simulink model "Messages1"  (R2020a)
settings: Solver=VariableStepAuto  StartTime=0.0  StopTime=0.3  RelTol=1e-3
settings Model: Creator=86188  LastModifiedBy=bzhan
settings DataIOCC: ReturnWorkspaceOutputs=off
settings DebuggingCC: ArithmeticOperatorsInVariantConditions=warning
settings SFSimCC: SimUseLocalCustomCode=off  CustomCodeUndefinedFunction=UseInterfaceOnly
settings RTWCC: RTWUseLocalCustomCode=off

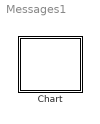
== system Messages1 ==
  Chart : Stateflow chart  TreatAsAtomicUnit=on

== stateflow chart Messages1/Chart ==
  state A
    en:
    f("en_A");
    M.data=3;
    send(M);
  state B
    en:
    f("en_B");
    y=1;
  state C
    en:
    f("en_C");
    y=2;
  (default) -> A
  B -> C : M
  A -> B : M[M.data==3]
  data: s function_input; M local
  function f(s):
    | function f(s)
    |   fprintf(s+"\n");
